simulink model "paper_matmul"  (R2017a)
settings: Solver=VariableStepAuto  StartTime=0.0  StopTime=10.0  RelTol=1e-3
libraries: ad_blocks x2
settings Model: Creator=eruffaldi  LastModifiedBy=eruffaldi

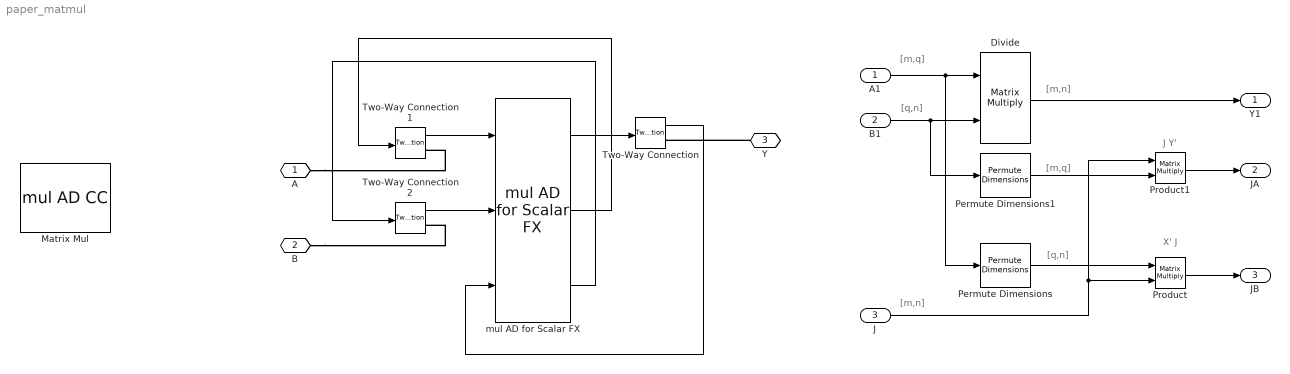
== system paper_matmul ==
  note: [q,n]
  note: [m,q]
  note: [m,n]
  note: X' J
  note: [m,q]
  note: J Y'
  note: [m,n]
  note: [q,n]
  A1 : Inport
  B1 : Inport  Port=2
  J : Inport  Port=3
  Divide : Product  Inputs=**  Multiplication=Matrix(*)
  Matrix Mul : ad_blocks/mul AD CC
  Permute Dimensions : PermuteDimensions
  Permute Dimensions1 : PermuteDimensions
  Product : Product  Multiplication=Matrix(*)
  Product1 : Product  Multiplication=Matrix(*)
  Two-Way Connection : TwoWayConnection
  Two-Way Connection1 : TwoWayConnection
  Two-Way Connection2 : TwoWayConnection
  mul AD for Scalar FX : ad_blocks/mul AD for Scalar FX
  A : PMIOPort  Port=1  Side=Left
  B : PMIOPort  Port=2  Side=Left
  Y : PMIOPort  Port=3  Side=Right
  Y1 : Outport
  JA : Outport  Port=2
  JB : Outport  Port=3
  wires:
  mul AD for Scalar FX/2 -> Two-Way Connection1/1
  mul AD for Scalar FX/1 -> Two-Way Connection/1
  Two-Way Connection1/1 -> mul AD for Scalar FX/1
  Two-Way Connection/1 -> mul AD for Scalar FX/3
  mul AD for Scalar FX/3 -> Two-Way Connection2/1
  Two-Way Connection2/1 -> mul AD for Scalar FX/2
  A1/1 -> Divide/1, Permute Dimensions/1
  Divide/1 -> Y1/1
  Product1/1 -> JA/1
  B1/1 -> Divide/2, Permute Dimensions1/1
  Permute Dimensions/1 -> Product/1
  J/1 -> Product/2, Product1/1
  Product/1 -> JB/1
  Permute Dimensions1/1 -> Product1/2
  connections:
  A/RConn1 -- Two-Way Connection1/RConn1
  B/RConn1 -- Two-Way Connection2/RConn1
  Y/RConn1 -- Two-Way Connection/RConn1
